simulink model "pendSim2"  (R2024a)
settings: Solver=FixedStepAuto  StartTime=0.0  StopTime=1  FixedStep=0.001  MaxStep=0.001  RelTol=1e-3
settings Model: Creator=mattf  LastModifiedBy=mattf

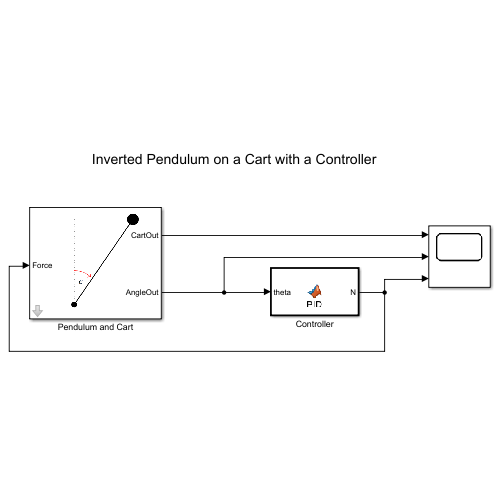
[thumbnail: Simulink's stored preview of the top-level diagram]
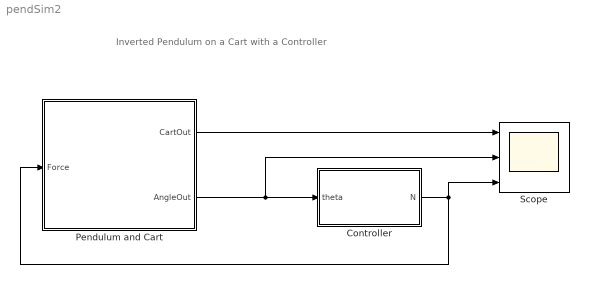
== system pendSim2 ==
  note: Inverted Pendulum on a Cart with a Controller
  Controller : MATLAB Function  TreatAsAtomicUnit=on  SystemSampleTime=0.001
  Pendulum and Cart : Subsystem  mask{Mcart=0.5, m=0.2, l=0.3/2, g=9.8, init=0.5236}
      mask prompts: Mcart "Cart Mass (kg):"; m "Pend Mass (kg):"; l "COM Distance (m):"; g "Acc due to Gravity (g):"; init "Initial Angle (rad):"
      mask Display: image('pen img.png');
  Scope : Scope  NumInputPorts=3
  wires:
  Pendulum and Cart/2(AngleOut) -> Scope/2, Controller/1(theta)
  Controller/1(N) -> Pendulum and Cart/1(Force), Scope/3
  Pendulum and Cart/1(CartOut) -> Scope/1

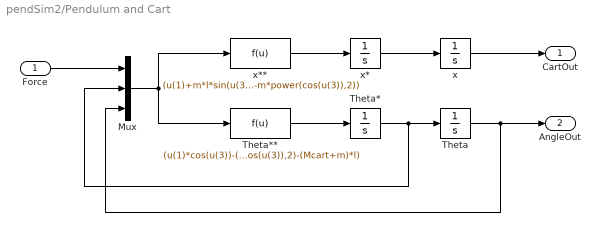
== system pendSim2/Pendulum and Cart ==
  Force : Inport
  Mux : Mux  Inputs=3
  Theta : Integrator  InitialCondition=init
  Theta* : Integrator
  Theta** : Fcn  Expr=(u(1)*cos(u(3))-(Mcart+m)*g*sin(u(3))+m*l*cos(u(3))*sin(u(3))*power(u(2),2))/(m*l*power(cos(u(3)),2)-(Mcart+m)*l)
  x : Integrator
  x* : Integrator
  x** : Fcn  Expr=(u(1)+m*l*sin(u(3))*power(u(2),2)-m*g*cos(u(3))*sin(u(3)))/(Mcart+m-m*power(cos(u(3)),2))
  CartOut : Outport
  AngleOut : Outport  Port=2
  wires:
  Mux/1 -> x**/1, Theta**/1
  x*/1 -> x/1
  x/1 -> CartOut/1
  Force/1 -> Mux/1
  Theta**/1 -> Theta*/1
  x**/1 -> x*/1
  Theta*/1 -> Mux/2, Theta/1
  Theta/1 -> Mux/3, AngleOut/1

== matlab function pendSim2/Controller ==
  settings: updateMethod=DISCRETE
  data: N output; theta input
function N = PID(theta)

    % call extrinsic python function
    coder.extrinsic('py.PIDController.PIDRun');

    % Call Python function and return result
    N = coder.nullcopy(zeros(1,1)); % no clue why, but this is need.
    N = double(py.PIDController.PIDRun(theta, 0.001));
    end
